simulink model "untitled1"  (R2018a)
settings: Solver=VariableStepAuto  StartTime=0.0  StopTime=10.0  RelTol=1e-3
libraries: pixhawk_slib_sensors_actuators x2, pixhawk_slib_uORB_RW x2
settings Model: Creator=Administrator  LastModifiedBy=Administrator

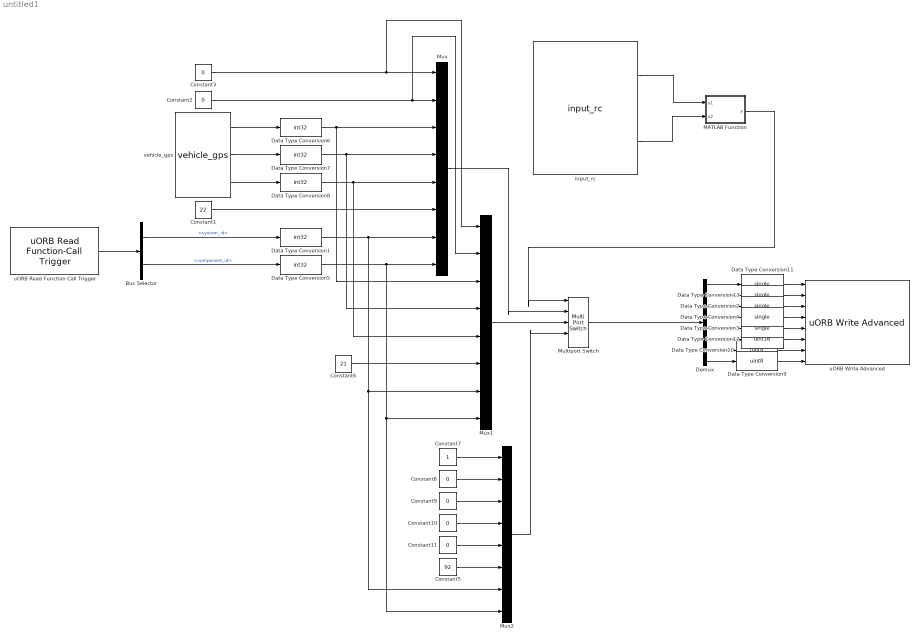
== system untitled1 ==
  Bus Selector : BusSelector  OutputSignals=system_id,component_id
  Constant1 : Constant  Value=22  OutDataTypeStr=int32
  Constant{2..3,8..11} (6 alike) : Constant  Value=0  OutDataTypeStr=int32
  Constant5 : Constant  Value=92  OutDataTypeStr=int32
  Constant6 : Constant  Value=21  OutDataTypeStr=int32
  Constant7 : Constant  OutDataTypeStr=int32
  Data Type Conversion{1,5..8} (5 alike) : DataTypeConversion  OutDataTypeStr=int32
  Data Type Conversion10 : DataTypeConversion  OutDataTypeStr=uint8
  Data Type Conversion{2..4,11,13} (5 alike) : DataTypeConversion  OutDataTypeStr=single
  Data Type Conversion12 : DataTypeConversion  OutDataTypeStr=uint16
  Data Type Conversion9 : DataTypeConversion  OutDataTypeStr=uint8
  Demux : Demux  Outputs=8
  MATLAB Function : MATLAB Function  TreatAsAtomicUnit=on
  Multiport Switch : MultiPortSwitch  Inputs=4
  Mux : Mux  Inputs=8
  Mux1 : Mux  Inputs=8
  Mux2 : Mux  Inputs=8
  input_rc : pixhawk_slib_sensors_actuators/input_rc  Description=|  sampletime=1/250  channel1=off  channel2=off  channel3=off  channel4=off  channel5=on  channel6=on  channel7=off  channel8=off  channel9=off  channel10=off  channel11=off  channel12=off  channel13=off  channel14=off  channel15=off  channel16=off  channel17=off  channel18=off  ch_count=off  rssi=off  rc_failsafe=off  rc_lost=off  rc_inputsource=off
      | RC Input Block
      | 
      | This block provides user input control to the model.
      | It uses the input_rc uORB topic.
      | 
      | The user has the ability to choose which channels are available as outputs from this block and also some optional outputs. These include 
      | Channels 1 through 18
      | double data type indicating the PWM value from the controller 
      | measured pulse widths for each of the supported channels 
      | Channel Count 
      | uint32 data type of the number of channels which are detector by the PX4 
      | RC Failsafe 
      | boolean data types indicating that the RC Tx is sending the FailSafe signal (if equipped and properly setup) 
      | explicit failsafe flag: true on TX failure or TX out of range , false otherwise. 
      | Only the true state is reliable, as there are some (PPM) receivers on the market going into failsafe without telling us explicitly. 
      | RC Input Source 
      | Enumeration data type indicating which source the RC input is from. 
      | Valid values are found in the ENUM file: RC_INPUT_SOURCE_ENUM.m 
      |           Enumeration members for class 'RC_INPUT_SOURCE_ENUM':
      |           RCINPUT_SOURCE_UNKNOWN         (0)
      |           RCINPUT_SOURCE_PX4FMU_PPM      (1)
      |           RCINPUT_SOURCE_PX4IO_PPM       (2)
      |           RCINPUT_SOURCE_PX4IO_SPEKTRUM  (3)
      |           RCINPUT_SOURCE_PX4IO_SBUS      (4)
      |           RCINPUT_SOURCE_PX4IO_ST24      (5)
      |           RCINPUT_SOURCE_MAVLINK         (6)
      |           RCINPUT_SOURCE_QURT            (7)
      |           RCINPUT_SOURCE_PX4FMU_SPEKTRUM (8)
      |           RCINPUT_SOURCE_PX4FMU_SBUS     (9)
      |           RCINPUT_SOURCE_PX4FMU_ST24     (10)
      |           RCINPUT_SOURCE_PX4FMU_SUMD     (11)
      |           RCINPUT_SOURCE_PX4FMU_DSM      (12)
      |           RCINPUT_SOURCE_PX4IO_SUMD      (13)
      | 
      | RSSI - Receive signal strength index 
      | receive signal strength indicator (RSSI): < 0: Undefined, 0: no signal, 255: full reception 
      | RC Lost Connection 
      | boolean data type indicating RC receiver connection status 
      | True, if no frame has arrived in the expected time, false otherwise. 
      | True usally means that the receiver has been disconnected, but can also indicate a radio link loss on "stupid" systems. 
      | Will remain false, if a RX with failsafe option continues to transmit frames after a link loss. 
      |   
      | Sample Model: px4demo_input_rc.slx
      settings: SourceProductName=Pixhawk Target Blocks
  uORB Read Function-Call Trigger : pixhawk_slib_uORB_RW/uORB Read Function-Call Trigger  uORB_Topic_str='vehicle_status'  BusObjVar=Bus: vehicle_status_SL  uORB_Interval=1  AsyncOutput=off  Fcn_call_select=Generate Function Call Signal  TaskName='Task1'  Poll_timeout=100  Ts=0.004
      settings: SourceProductName=Pixhawk Target Blocks
  uORB Write Advanced : pixhawk_slib_uORB_RW/uORB Write Advanced  Ts=0  uORB_AdvtQueue=on  uORB_FieldEnabledArr="0  0  0  1  0  0  0  0  0  0  0"  uORB_Topic_str=0  uORB_Struct_DT="[1  1  1  1  1]"  BlockInputCount=5  uORB_StructParams="[\"voltage_v\",\"voltage_filtered_v\",\"current_a\",\"current_filtered_a\",\"remaining\"]"  uORB_PortSizes="[1  1  1  1]"  MsgSizeOf=0  MW_update=true
      settings: SourceProductName=Pixhawk Target Blocks
  vehicle_gps : pixhawk_slib_sensors_actuators/vehicle_gps  Description=|  sampletime=1/250  show_alt=on  show_ts_gps=off  show_vel=off  show_fixtype=off  show_numsat=off
      | This block will provide GPS signals from the uORB topic publisher: vehicle_gps_position.  
      | You must ensure that you have the gps topic executed as part of the start-up script in order to get valid signal values. 
      | Refer to the sample model: px4demo_gps.slx 
      | Signal definitions: 
      | Latitude – (int32) global coordinate given in 1e-7 degrees 
      | Longitude – (int32) global coordinate given in 1e-7 degrees 
      | Position TS – (double) timestamp for position information 
      | Altitude – (int32) in 1e-3 meters (millimeters) above MSL (mean sea level) 
      | GPS TS – (double) timestamp (microseconds in GPS format).  This is the timestamp that comes from the GPS module. 
      | Velocity TS – (single) timestamp for velocity information 
      | Velocity – (single) GPS ground speed in meters/second 
      | GPS Fix Type – (uint8) 0-1 = No fix, 2 = 2D fix, 3= 3D fix 
      | Num Satellites – (uint8) the number of satellites used in calculations
      settings: SourceProductName=Pixhawk Target Blocks
  wires:
  Constant8/1 -> Mux2/2
  Data Type Conversion6/1 -> Mux1/3, Mux/3
  Constant7/1 -> Mux2/1
  Constant9/1 -> Mux2/3
  input_rc/2 -> MATLAB Function/2(u2)
  Demux/3 -> Data Type Conversion2/1
  Constant11/1 -> Mux2/5
  Multiport Switch/1 -> Demux/1
  Demux/8 -> Data Type Conversion9/1
  Constant1/1 -> Mux/6
  Demux/4 -> Data Type Conversion4/1
  Constant10/1 -> Mux2/4
  uORB Read Function-Call Trigger/1 -> Bus Selector/1
  Mux2/1 -> Multiport Switch/4
  input_rc/1 -> MATLAB Function/1(u1)
  Data Type Conversion12/1 -> uORB Write Advanced/6
  Demux/7 -> Data Type Conversion10/1
  Data Type Conversion2/1 -> uORB Write Advanced/3
  MATLAB Function/1(y) -> Multiport Switch/1
  Data Type Conversion4/1 -> uORB Write Advanced/4
  Mux/1 -> Multiport Switch/2
  Constant3/1 -> Mux/1, Mux1/1
  Demux/5 -> Data Type Conversion3/1
  Data Type Conversion10/1 -> uORB Write Advanced/7
  Demux/1 -> Data Type Conversion11/1
  vehicle_gps/3 -> Data Type Conversion8/1
  Data Type Conversion1/1 -> Mux2/7, Mux1/7, Mux/7
  Data Type Conversion9/1 -> uORB Write Advanced/8
  Constant6/1 -> Mux1/6
  Data Type Conversion5/1 -> Mux2/8, Mux1/8, Mux/8
  Data Type Conversion7/1 -> Mux1/4, Mux/4
  Data Type Conversion13/1 -> uORB Write Advanced/2
  vehicle_gps/1 -> Data Type Conversion6/1
  Constant2/1 -> Mux/2, Mux1/2
  Data Type Conversion8/1 -> Mux1/5, Mux/5
  Demux/2 -> Data Type Conversion13/1
  Data Type Conversion3/1 -> uORB Write Advanced/5
  vehicle_gps/2 -> Data Type Conversion7/1
  Bus Selector/1 -> Data Type Conversion1/1  "<system_id>"
  Bus Selector/2 -> Data Type Conversion5/1  "<component_id>"
  Constant5/1 -> Mux2/6
  Data Type Conversion11/1 -> uORB Write Advanced/1
  Demux/6 -> Data Type Conversion12/1
  Mux1/1 -> Multiport Switch/3

== matlab function untitled1/MATLAB Function ==
  data: u1 input; y output; u2 input
function y = fcn(u1,u2)
y=4;
persistent i;
if isempty(i)
   i=0;
end
persistent j;
if isempty(j)
   j=0;
end
persistent k;
if isempty(k)
   k=0;
end
if((u1<=1200)&i<=1)
    y=1;
    i=i+1;
    j=0;
    k=0;

end
if((1600<=u1)&j<=1)
    y=2;
    j=j+1;
    i=0;
    k=0;

end
if((1500<=u2)&k<=1)
    y=3;
    k=k+1;
    i=0;
    j=0;
end
end
